simulink subsystem "Controller_Wind_H2"  (R2022a)
settings: Solver=VariableStepAuto  StartTime=0.0  StopTime=10.0  RelTol=1e-3
undefined symbols (not defined in the file or in its folder): Setpoint
libraries: nesl_utility x7, slpidlib x1, simulink x1, spsPWMGenerator2LevelLib x1, ee_lib x1, spsPLL3phLib x1, spsRMSLib x1, fl_lib x1
settings Model: Creator=jsagardu  LastModifiedBy=jsagardu
settings DebuggingCC: UnconnectedInputMsg=warning  UnconnectedOutputMsg=warning  UnconnectedLineMsg=warning
settings RTWCC: DLArmComputeVersion=19.05

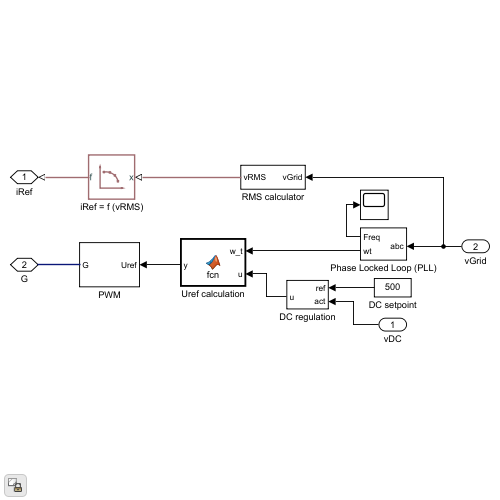
[thumbnail: Simulink's stored preview of the top-level diagram]
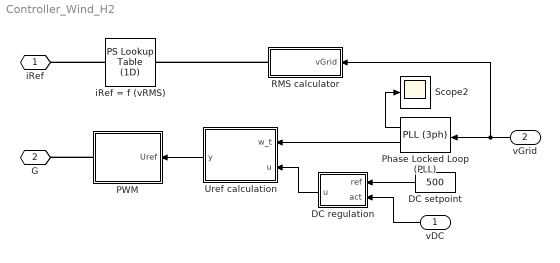
== system Controller_Wind_H2 ==
  vDC : Inport
  vGrid : Inport  Port=2
  DC regulation : Subsystem
  DC setpoint : Constant  Value=500
  PWM : Subsystem
  "Phase Locked Loop (PLL) " : spsPLL3phLib/PLL (3ph)  Fmin=15  Par_Init=[0, 50]  ParK=[180, 3200, 1]  TcD=PLL.Tc_Derivative  MaxRateChangeFreq=PLL.Max_Rate_Freq  FilterCutOffFreq=7.5  Ts=0  AGC=on
  RMS calculator : Subsystem
  Scope2 : Scope
  Uref calculation : MATLAB Function  TreatAsAtomicUnit=on
  iRef = f (vRMS) : fl_lib/Physical Signals/Lookup Tables/PS Lookup Table (1D)  x=Setpoint.AC.Vrms_vect V  f=Setpoint.AC.Ie_vect A  interp_method=simscape.enum.interpolation.linear  extrap_method=simscape.enum.extrapolation.nearest
      settings: SourceProductBaseCode=PW,SS,VE
  iRef : PMIOPort  Side=Right
  G : PMIOPort  Port=2  Side=Right
  wires:
  Uref calculation/1(y) -> PWM/1(Uref)
  vGrid/1 -> "Phase Locked Loop (PLL) "/1, RMS calculator/1(vGrid)
  "Phase Locked Loop (PLL) "/1 -> Scope2/1
  "Phase Locked Loop (PLL) "/2 -> Uref calculation/1(w_t)
  DC setpoint/1 -> DC regulation/1(ref)
  DC regulation/1(u) -> Uref calculation/2(u)
  vDC/1 -> DC regulation/2(act)
  connections:
  iRef = f (vRMS)/RConn1 -- iRef/RConn1
  PWM/RConn1 -- G/RConn1
  RMS calculator/RConn1 -- iRef = f (vRMS)/LConn1

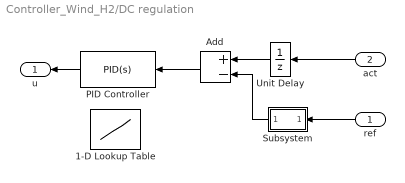
== system Controller_Wind_H2/DC regulation ==
  ref : Inport
  act : Inport  Port=2
  1-D Lookup Table : Lookup_n-D  NumberOfTableDimensions=1  BreakpointsForDimension1=[475 530 683 887.5]  Table=[1 0.75 0.625 0.5]  InternalRulePriority=Speed  RndMeth=Simplest
  Add : Sum  Inputs=+-
  PID Controller : slpidlib/PID Controller  Controller=PID  Form=Parallel  TimeDomain=Continuous-time  UseExternalTs=off  SampleTime=-1  IntegratorMethod=Forward Euler  FilterMethod=Forward Euler  ControllerParametersSource=internal  P=5  I=1  UseKiTs=off  D=0  N=100  UseFilter=on  TunerSelectOption=Transfer Function Based (PID Tuner App)  InitialConditionSource=internal  InitialConditionForIntegrator=0  InitialConditionForFilter=0  DifferentiatorICPrevScaledInput=0  ExternalReset=none  TrackingMode=off  Kt=1  LimitOutput=on  SatLimitsSource=internal  UpperSaturationLimit=2  LowerSaturationLimit=0  LinearizeAsGain=on  AntiWindupMode=none  Kb=1  POutMin=[]  POutMax=[]  IOutMin=[]  IOutMax=[]  DOutMin=[]  DOutMax=[]  NOutMin=[]  NOutMax=[]  SumOutMin=[]  SumOutMax=[]  SaturationOutMin=[]  SaturationOutMax=[]  PParamMin=[]  PParamMax=[]  IParamMin=[]  IParamMax=[]  DParamMin=[]  DParamMax=[]  NParamMin=[]  NParamMax=[]  KbParamMin=[]  KbParamMax=[]  KtParamMin=[]  KtParamMax=[]  KbOutMin=[]  KbOutMax=[]  KtOutMin=[]  KtOutMax=[]  IntegratorOutMin=[]  IntegratorOutMax=[]  FilterOutMin=[]  FilterOutMax=[]  SumI1OutMin=[]  SumI1OutMax=[]  SumI2OutMin=[]  SumI2OutMax=[]  SumI3OutMin=[]  SumI3OutMax=[]  SumI4OutMin=[]  SumI4OutMax=[]  SumDOutMin=[]  SumDOutMax=[]  DifferentiatorOutMin=[]  DifferentiatorOutMax=[]  FilterDiffOutCoefMin=[]  FilterDiffOutCoefMax=[]  ReciprocalOutMin=[]  ReciprocalOutMax=[]  SumDenOutMin=[]  SumDenOutMax=[]  SumNumOutMin=[]  SumNumOutMax=[]  DivideOutMin=[]  DivideOutMax=[]  UdiffTsProdOutMin=[]  UdiffTsProdOutMax=[]  NTsProdOutMin=[]  NTsProdOutMax=[]  UintegralTsProdOutMin=[]  UintegralTsProdOutMax=[]  UngainTsProdOutMin=[]  UngainTsProdOutMax=[]  IntegratorContinuousStateAttributes=''  IntegratorStateMustResolveToSignalObject=off  IntegratorRTWStateStorageClass=Auto  FilterContinuousStateAttributes=''  FilterStateMustResolveToSignalObject=off  FilterRTWStateStorageClass=Auto  ParallelPVariant=InternalParameters  IdealPVariant=Disabled  IVariant=InternalParameters  DVariant=InternalParameters  IntegratorVariant=Continuous  SatVariant=Enabled  AWVariant=Passthrough  PCopyVariant=Disabled  TRVariant=Disabled  FdbkBlocksVariant=Forward  IdealPFdbkVariant=Disabled  SatFdbkVariant=Disabled  DerivativeFilterVariant=ContFilter  NVariant=InternalParameters  NCopyVariant=Disabled  FilterICVariant=InternalICsFilter  IntegratorICVariant=InternalICs  ExternalResetVariant=Disabled  TRSumVariant=Passthrough  SumFdbkVariant=Disabled  SumVariant=Sum_PID  TsampFilterVariant=InternalTs  TsampNgainVariant=Passthrough  TsampIntegralVariant=Passthrough  ExternalSaturationOutDataTypeStr=Inherit: Same as second input  aMode=0
  Subsystem : Subsystem
  Unit Delay : UnitDelay  SampleTime=-1  HasFrameUpgradeWarning=on
  u : Outport
  wires:
  Subsystem/1(Out1) -> Add/2
  ref/1 -> Subsystem/1(In1)
  Unit Delay/1 -> Add/1
  PID Controller/1 -> u/1
  act/1 -> Unit Delay/1
  Add/1 -> PID Controller/1

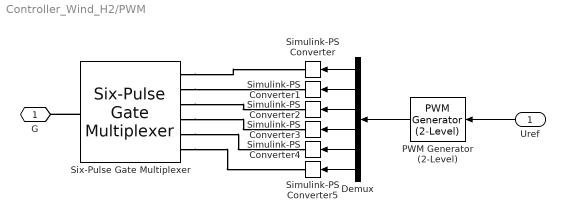
== system Controller_Wind_H2/PWM ==
  Uref : Inport
  Demux : Demux  Outputs=6
  PWM Generator (2-Level) : spsPWMGenerator2LevelLib/PWM Generator (2-Level)  ModulatorType=Three-phase bridge (6 pulses)  ModulatorMode=Unsynchronized  Fc=Setpoint.AC.Fsw  Pc=0  nF=27  MinMax="[ -1  1 ]"  SamplingTechnique=Natural  ModulatingSignals=off  m=0.8  Freq=450  Phase=0  Ts=Setpoint.AC.ts  ShowCarrierOutport=off
  Simulink-PS Converter{,1..5} (6 alike) : nesl_utility/Simulink-PS Converter  PhysicalDomain=network_engine_domain  SubClassName=ps_input  LeftPortType=input  RightPortType=output  PseudoPeriodic=off  Frequencies=[]  NoiseDistribution=none  NoiseParameters=[]  Unit=1  AffineConversion=off  FilteringAndDerivatives=provide  SimscapeFilterOrder=1  InputFilterTimeConstant=0.001  UdotUserProvided=0
      settings: SourceProductBaseCode=SS,PW,VE
  Six-Pulse Gate Multiplexer : ee_lib/Semiconductors & Converters/Converters/Six-Pulse Gate Multiplexer  port_option=ee.enum.controlport.ps
      settings: SourceProductBaseCode=PS
  G : PMIOPort  Side=Right
  wires:
  Demux/6 -> Simulink-PS Converter5/1
  Demux/1 -> Simulink-PS Converter/1
  PWM Generator (2-Level)/1 -> Demux/1
  Demux/4 -> Simulink-PS Converter3/1
  Demux/3 -> Simulink-PS Converter2/1
  Uref/1 -> PWM Generator (2-Level)/1
  Demux/5 -> Simulink-PS Converter4/1
  Demux/2 -> Simulink-PS Converter1/1
  connections:
  Six-Pulse Gate Multiplexer/RConn1 -- G/RConn1
  Six-Pulse Gate Multiplexer/LConn4 -- Simulink-PS Converter3/RConn1
  Six-Pulse Gate Multiplexer/LConn1 -- Simulink-PS Converter/RConn1
  Six-Pulse Gate Multiplexer/LConn5 -- Simulink-PS Converter4/RConn1
  Six-Pulse Gate Multiplexer/LConn6 -- Simulink-PS Converter5/RConn1
  Six-Pulse Gate Multiplexer/LConn3 -- Simulink-PS Converter2/RConn1
  Six-Pulse Gate Multiplexer/LConn2 -- Simulink-PS Converter1/RConn1

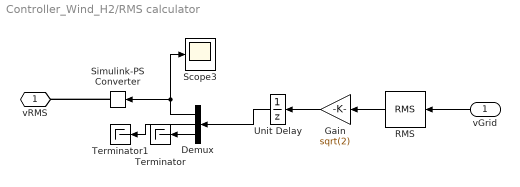
== system Controller_Wind_H2/RMS calculator ==
  vGrid : Inport
  Demux : Demux  Outputs=3
  Gain : Gain  Gain=sqrt(2)
  RMS : spsRMSLib/RMS  TrueRMS=on  Freq=5  RMSInit=230/sqrt(2)  Ts=0
  Scope3 : Scope
  Simulink-PS Converter : nesl_utility/Simulink-PS Converter  PhysicalDomain=network_engine_domain  SubClassName=ps_input  LeftPortType=input  RightPortType=output  PseudoPeriodic=off  Frequencies=[]  NoiseDistribution=none  NoiseParameters=[]  Unit=V  AffineConversion=off  FilteringAndDerivatives=filter  SimscapeFilterOrder=1  InputFilterTimeConstant=0.1  UdotUserProvided=0
      settings: SourceProductBaseCode=SS,PW,VE
  Terminator : Terminator
  Terminator1 : Terminator
  Unit Delay : UnitDelay  InitialCondition=230  SampleTime=-1  HasFrameUpgradeWarning=on
  vRMS : PMIOPort  Side=Right
  wires:
  vGrid/1 -> RMS/1
  Demux/3 -> Terminator/1
  Unit Delay/1 -> Demux/1
  Gain/1 -> Unit Delay/1
  RMS/1 -> Gain/1
  Demux/2 -> Terminator1/1
  Demux/1 -> Scope3/1, Simulink-PS Converter/1
  connections:
  Simulink-PS Converter/RConn1 -- vRMS/RConn1

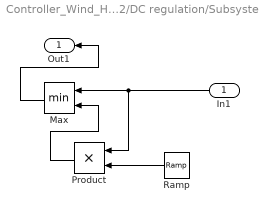
== system Controller_Wind_H2/DC regulation/Subsystem ==
  In1 : Inport
  Max : MinMax  Inputs=2
  Product : Product
  Ramp : simulink/Sources/Ramp  slope=1/0.5  start=0  InitialOutput=0
  Out1 : Outport
  wires:
  Product/1 -> Max/2
  In1/1 -> Max/1, Product/1
  Max/1 -> Out1/1
  Ramp/1 -> Product/2

== matlab function Controller_Wind_H2/Uref calculation ==
  data: w_t input; u input; y output
function y = fcn(w_t, u)

ya = u*sin(w_t+0);
yb = u*sin(w_t-2*pi/3);
yc = u*sin(w_t+2*pi/3);

y = [ya yb yc]';
